simulink model "Suspension_System"  (R2019a)
settings: Solver=VariableStepAuto  StartTime=0.0  StopTime=50  RelTol=1e-3
settings Model: Creator=Dear User  LastModifiedBy=Dear User

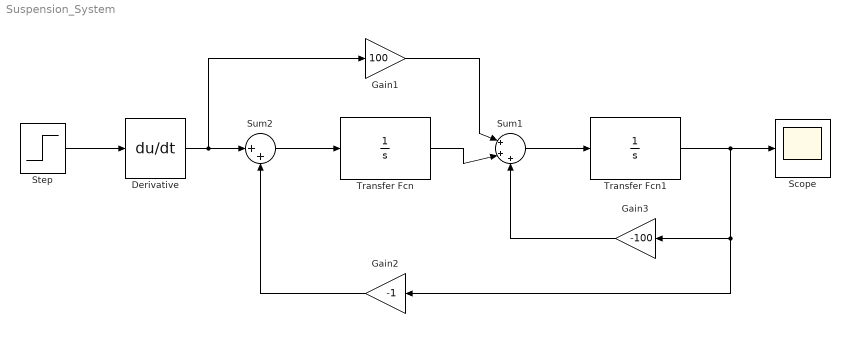
== system Suspension_System ==
  Derivative : Derivative
  Gain1 : Gain  Gain=100
  Gain2 : Gain  Gain=-1
  Gain3 : Gain  Gain=-100
  Scope : Scope
  Step : Step  Time=0.001  SampleTime=0
  Sum1 : Sum  Inputs=|+++
  Sum2 : Sum  Inputs=|++
  Transfer Fcn : TransferFcn  Denominator=[1 0]
  Transfer Fcn1 : TransferFcn  Denominator=[1 0]
  wires:
  Sum2/1 -> Transfer Fcn/1
  Sum1/1 -> Transfer Fcn1/1
  Transfer Fcn1/1 -> Gain2/1, Gain3/1, Scope/1
  Gain3/1 -> Sum1/3
  Transfer Fcn/1 -> Sum1/2
  Gain1/1 -> Sum1/1
  Step/1 -> Derivative/1
  Derivative/1 -> Gain1/1, Sum2/1
  Gain2/1 -> Sum2/2
